simulink model "PTSD_single_channel_local_min_max_2"  (R2019b)
settings: Solver=VariableStepAuto  StartTime=0.0  StopTime=10  RelTol=1e-3
libraries: simulink x10, dspstat3 x7, dspswit3 x1
settings Model: Creator=sbuccelli  LastModifiedBy=sbuccelli

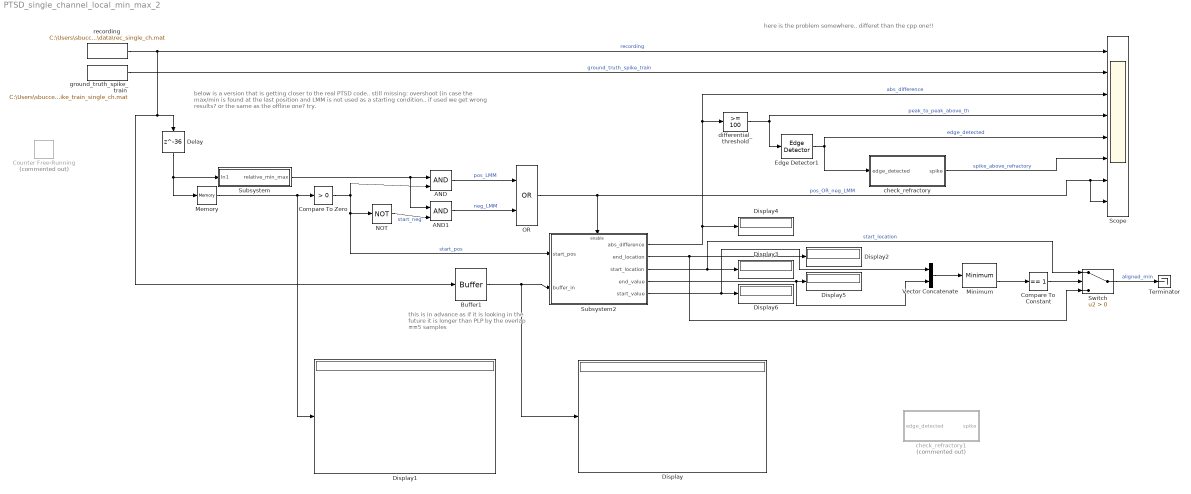
== system PTSD_single_channel_local_min_max_2 ==
  note: here is the problem somewhere.. differet than the cpp one!!
  note: below is a version that is getting closer to the real PTSD code..
      | still missing: overshoot (in case the max/min is found at the last position and LMM is not used as a starting condition.. if used we get wrong results? or the same as the offline one? try.
  note: this is in advance as if it is looking in the future
      | it is longer than PLP by the overlap ==5 samples
  AND : Logic  IconShape=distinctive  AllPortsSameDT=off  OutDataTypeStr=boolean
  AND1 : Logic  IconShape=distinctive  AllPortsSameDT=off  OutDataTypeStr=boolean
  Buffer1 : Buffer  N=38  V=37  OutputFrames=off
  Compare To Constant : simulink/Logic and Bit Operations/Compare To Constant  relop===  const=1  OutDataTypeStr=boolean
  Compare To Zero : simulink/Logic and Bit Operations/Compare To Zero  relop=>  OutDataTypeStr=boolean
  Counter Free-Running : simulink/Sources/Counter Free-Running  Commented=on  NumBits=32  tsamp=-1
  Delay : Delay  DelayLength=36
  Display{,1..6} (7 alike) : Display
  Edge Detector1 : dspswit3/Edge Detector  InputProcessing=Columns as channels (frame based)
      settings: SourceProductName=DSP System Toolbox  SourceProductBaseCode=DS
  Memory : Memory  InheritSampleTime=on
  Minimum : dspstat3/Minimum  operation=minimum  fcn=Value and Index  indexBase=One  operateOver=Each column  Dimension=1  InputProcessing=Columns as channels (frame based)  reset=None  roiEnable=off  roiType=Rectangles  roiPortion=Entire ROI  roiOutput=Individual statistics for each ROI  roiFlag=off  roundingMode=Floor  overflowMode=off
      settings: SourceProductName=DSP System Toolbox  SourceProductBaseCode=DS
  NOT : Logic  Operator=NOT  IconShape=distinctive  AllPortsSameDT=off  OutDataTypeStr=boolean
  OR : Logic  Operator=OR  IconShape=distinctive  AllPortsSameDT=off  OutDataTypeStr=boolean
  Scope : Scope  NumInputPorts=8
  Subsystem : Subsystem
  Subsystem2 : Subsystem
  Switch : Switch  Criteria=u2 > Threshold
  Terminator : Terminator
  Vector Concatenate : Concatenate
  check_refractory : Subsystem
  check_refractory1 : Subsystem  Commented=on
  differential_threshold : simulink/Logic and Bit Operations/Compare To Constant  relop=>=  const=100  OutDataTypeStr=boolean
  ground_truth_spike_train : FromFile  FileName=C:\Users\sbuccelli\Documents\GitHub\closed-loop-neuroscience\data\spike_train_single_ch.mat  SampleTime=1/32e3
  recording : FromFile  FileName=C:\Users\sbuccelli\Documents\GitHub\closed-loop-neuroscience\data\rec_single_ch.mat  SampleTime=1/32e3
  wires:
  recording/1 -> Buffer1/1, Delay/1, Scope/1  "recording"
  ground_truth_spike_train/1 -> Scope/2  "ground_truth_spike_train"
  Subsystem/1(relative_min_max) -> AND/1, AND1/1
  Compare To Zero/1 -> Subsystem2/1(start_pos), NOT/1, AND/2  "start_pos"
  NOT/1 -> AND1/2  "start_neg"
  AND/1 -> OR/1  "pos_LMM"
  AND1/1 -> OR/2  "neg_LMM"
  OR/1 -> Scope/7, Scope/8, Subsystem2/Enable  "pos_OR_neg_LMM"
  Delay/1 -> Memory/1, Subsystem/1(In1)
  differential_threshold/1 -> Scope/4, Edge Detector1/1  "peak_to_peak_above_th"
  Subsystem2/1(abs_difference) -> Display4/1, Scope/3, differential_threshold/1  "abs_difference"
  Buffer1/1 -> Display/1, Subsystem2/2(buffer_in)
  Edge Detector1/1 -> check_refractory/1(edge_detected), Scope/5  "edge_detected"
  check_refractory/1(spike) -> Scope/6  "spike_above_refractory"
  Memory/1 -> Display1/1, Compare To Zero/1
  Subsystem2/2(end_location) -> Switch/3, Display2/1
  Subsystem2/4(end_value) -> Vector Concatenate/2, Display5/1
  Subsystem2/5(start_value) -> Vector Concatenate/1, Display6/1
  Subsystem2/3(start_location) -> Switch/1, Display3/1  "start_location"
  Vector Concatenate/1 -> Minimum/1
  Minimum/2 -> Compare To Constant/1
  Compare To Constant/1 -> Switch/2
  Switch/1 -> Terminator/1  "aligned_min"

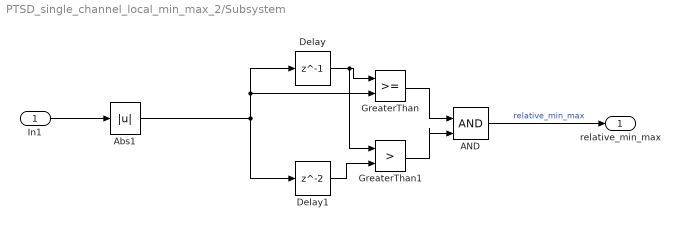
== system PTSD_single_channel_local_min_max_2/Subsystem ==
  In1 : Inport
  AND : Logic  IconShape=distinctive  AllPortsSameDT=off  OutDataTypeStr=boolean
  Abs1 : Abs
  Delay : Delay  DelayLength=1
  Delay1 : Delay
  GreaterThan : RelationalOperator  OutDataTypeStr=boolean  RndMeth=Simplest
  GreaterThan1 : RelationalOperator  Operator=>  OutDataTypeStr=boolean  RndMeth=Simplest
  relative_min_max : Outport
  wires:
  In1/1 -> Abs1/1
  Delay1/1 -> GreaterThan1/2
  GreaterThan1/1 -> AND/2
  GreaterThan/1 -> AND/1
  Delay/1 -> GreaterThan1/1, GreaterThan/1
  AND/1 -> relative_min_max/1  "relative_min_max"
  Abs1/1 -> Delay/1, GreaterThan/2, Delay1/1

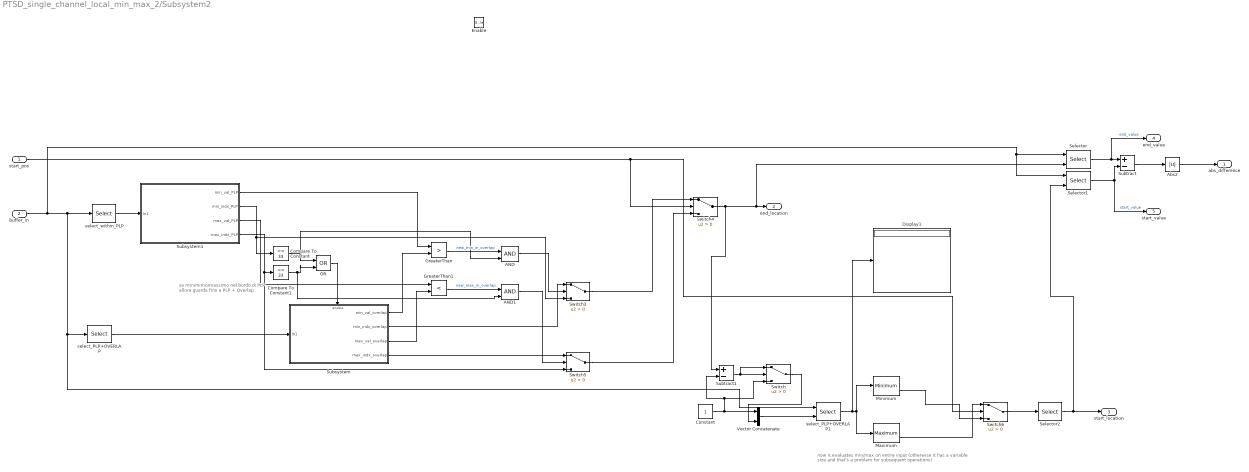
== system PTSD_single_channel_local_min_max_2/Subsystem2 ==
  note: now it evaluates min/max on entire input (otherwise it has a variable size and that's a problem for subsequent operations)
  note: se minimimo/massimo nel bordo di PLP allora guarda fino a PLP + Overlap
  start_pos : Inport
  buffer_in : Inport  Port=2
  Enable : EnablePort  PropagateVarSize=During execution
  AND : Logic  IconShape=distinctive  AllPortsSameDT=off  OutDataTypeStr=boolean
  AND1 : Logic  IconShape=distinctive  AllPortsSameDT=off  OutDataTypeStr=boolean
  Abs2 : Abs
  Compare To Constant : simulink/Logic and Bit Operations/Compare To Constant  relop===  const=33  OutDataTypeStr=boolean
  Compare To Constant1 : simulink/Logic and Bit Operations/Compare To Constant  relop===  const=33  OutDataTypeStr=boolean
  Constant : Constant
  Display1 : Display
  GreaterThan : RelationalOperator  Operator=>  OutDataTypeStr=boolean  RndMeth=Simplest
  GreaterThan1 : RelationalOperator  Operator=<  OutDataTypeStr=boolean  RndMeth=Simplest
  Maximum : dspstat3/Maximum  operation=maximum  fcn=Value and Index  indexBase=One  operateOver=Entire input  Dimension=1  InputProcessing=Columns as channels (frame based)  reset=None  roiEnable=off  roiType=Rectangles  roiPortion=Entire ROI  roiOutput=Individual statistics for each ROI  roiFlag=off  roundingMode=Floor  overflowMode=off  accumDataTypeStr=Inherit: Same as product output  accumLastDataTypeStr=Inherit: Same as product output
  Minimum : dspstat3/Minimum  operation=minimum  fcn=Value and Index  indexBase=One  operateOver=Entire input  Dimension=1  InputProcessing=Columns as channels (frame based)  reset=None  roiEnable=off  roiType=Rectangles  roiPortion=Entire ROI  roiOutput=Individual statistics for each ROI  roiFlag=off  roundingMode=Floor  overflowMode=off
      settings: SourceProductName=DSP System Toolbox  SourceProductBaseCode=DS
  OR : Logic  Operator=OR  IconShape=distinctive  AllPortsSameDT=off  OutDataTypeStr=boolean
  Selector : Selector  IndexOptions=Index vector (port)  Indices=[1 3]  OutputSizes=1
  Selector1 : Selector  IndexOptions=Index vector (port)  Indices=[1 3]  OutputSizes=1
  Selector2 : Selector  NumberOfDimensions=2  IndexOptions=Select all,Index vector (dialog)  Indices=[1 3],1  OutputSizes=1,1
  Subsystem : Subsystem
  Subsystem1 : Subsystem
  Subtract : Sum  Inputs=+-
  Subtract1 : Sum  Inputs=+-
  Switch{,3..6} (5 alike) : Switch  Criteria=u2 > Threshold
  Vector Concatenate : Concatenate
  select_PLP+OVERLAP : Selector  NumberOfDimensions=2  InputPortWidth=3  IndexOptions=Index vector (dialog),Index vector (dialog)  Indices=[34:38],1  OutputSizes=1,1
  select_PLP+OVERLAP1 : Selector  NumberOfDimensions=2  InputPortWidth=3  IndexOptions=Starting and ending indices (port),Index vector (dialog)  Indices=[25:29],1  OutputSizes=1,1
  select_within_PLP : Selector  NumberOfDimensions=2  InputPortWidth=3  IndexOptions=Index vector (dialog),Index vector (dialog)  Indices=[1:33],1  OutputSizes=1,1
  abs_difference : Outport
  end_location : Outport  Port=2
  start_location : Outport  Port=3
  end_value : Outport  Port=4
  start_value : Outport  Port=5
  wires:
  Abs2/1 -> abs_difference/1
  buffer_in/1 -> Selector1/1, Selector/1, select_within_PLP/1, select_PLP+OVERLAP1/1, select_PLP+OVERLAP/1
  Subtract/1 -> Abs2/1
  Compare To Constant/1 -> OR/1, AND/2
  Compare To Constant1/1 -> AND1/2, OR/2
  OR/1 -> Subsystem/Enable
  select_PLP+OVERLAP/1 -> Subsystem/1(In1)
  select_within_PLP/1 -> Subsystem1/1(In1)
  Subsystem1/2(min_indx_PLP) -> Switch3/3, Compare To Constant/1
  Subsystem1/4(max_indx_PLP) -> Switch5/3, Compare To Constant1/1
  Subsystem1/1(min_val_PLP) -> GreaterThan/1
  Subsystem/1(min_val_overlap) -> GreaterThan/2
  Subsystem1/3(max_val_PLP) -> GreaterThan1/1
  Subsystem/3(max_val_overlap) -> GreaterThan1/2
  GreaterThan/1 -> AND/1  "new_min_in_overlap"
  GreaterThan1/1 -> AND1/1  "new_max_in_overlap"
  AND/1 -> Switch3/2
  AND1/1 -> Switch5/2
  Switch3/1 -> Switch4/1
  Switch5/1 -> Switch4/3
  Subsystem/2(min_indx_overlap) -> Switch3/1
  Subsystem/4(max_indx_overlap) -> Switch5/1
  Vector Concatenate/1 -> select_PLP+OVERLAP1/2
  start_pos/1 -> Switch4/2, Switch6/2
  select_PLP+OVERLAP1/1 -> Display1/1, Maximum/1, Minimum/1
  Minimum/2 -> Switch6/3
  Maximum/2 -> Switch6/1
  Selector/1 -> end_value/1, Subtract/1  "end_value"
  Selector1/1 -> start_value/1, Subtract/2  "start_value"
  Switch4/1 -> Selector/2, end_location/1, Subtract1/1
  Switch6/1 -> Selector2/1
  Selector2/1 -> start_location/1, Selector1/2
  Subtract1/1 -> Switch/1, Switch/2
  Constant/1 -> Vector Concatenate/1, Switch/3, Subtract1/2
  Switch/1 -> Vector Concatenate/2

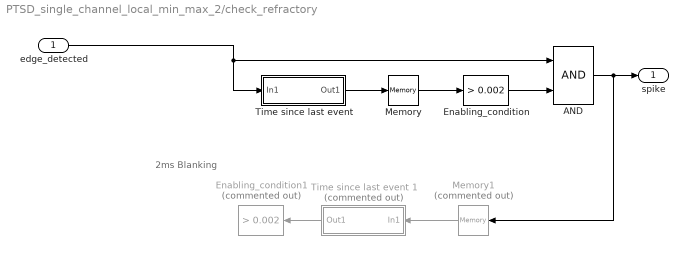
== system PTSD_single_channel_local_min_max_2/check_refractory ==
  note: 2ms Blanking
  edge_detected : Inport
  AND : Logic  IconShape=distinctive  AllPortsSameDT=off  OutDataTypeStr=boolean
  Enabling_condition : simulink/Logic and Bit Operations/Compare To Constant  relop=>  const=0.002  OutDataTypeStr=boolean
  Enabling_condition1 : simulink/Logic and Bit Operations/Compare To Constant  Commented=on  relop=>  const=0.002  OutDataTypeStr=boolean
  Memory : Memory  InheritSampleTime=on
  Memory1 : Memory  Commented=on  InheritSampleTime=on
  "Time since last event " : Subsystem
  Time since last event 1 : Subsystem  Commented=on
  spike : Outport
  wires:
  Enabling_condition/1 -> AND/2
  Memory/1 -> Enabling_condition/1
  "Time since last event "/1(Out1) -> Memory/1
  AND/1 -> Memory1/1, spike/1
  Time since last event 1/1(Out1) -> Enabling_condition1/1
  edge_detected/1 -> "Time since last event "/1(In1), AND/1
  Memory1/1 -> Time since last event 1/1(In1)

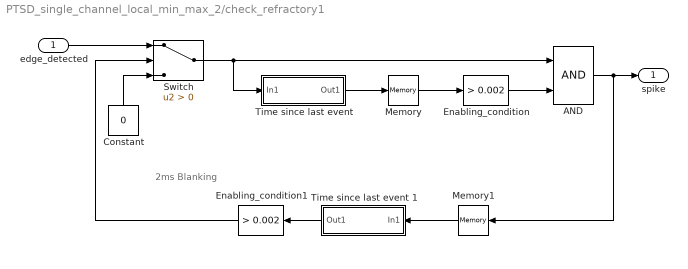
== system PTSD_single_channel_local_min_max_2/check_refractory1 ==
  note: 2ms Blanking
  edge_detected : Inport
  AND : Logic  IconShape=distinctive  AllPortsSameDT=off  OutDataTypeStr=boolean
  Constant : Constant  Value=0  SampleTime=-1
  Enabling_condition : simulink/Logic and Bit Operations/Compare To Constant  relop=>  const=0.002  OutDataTypeStr=boolean
  Enabling_condition1 : simulink/Logic and Bit Operations/Compare To Constant  relop=>  const=0.002  OutDataTypeStr=boolean
  Memory : Memory  InheritSampleTime=on
  Memory1 : Memory  InheritSampleTime=on
  Switch : Switch  Criteria=u2 > Threshold
  "Time since last event " : Subsystem
  Time since last event 1 : Subsystem
  spike : Outport
  wires:
  Enabling_condition/1 -> AND/2
  Memory/1 -> Enabling_condition/1
  "Time since last event "/1(Out1) -> Memory/1
  AND/1 -> Memory1/1, spike/1
  Time since last event 1/1(Out1) -> Enabling_condition1/1
  edge_detected/1 -> Switch/1
  Constant/1 -> Switch/3
  Switch/1 -> "Time since last event "/1(In1), AND/1
  Memory1/1 -> Time since last event 1/1(In1)
  Enabling_condition1/1 -> Switch/2

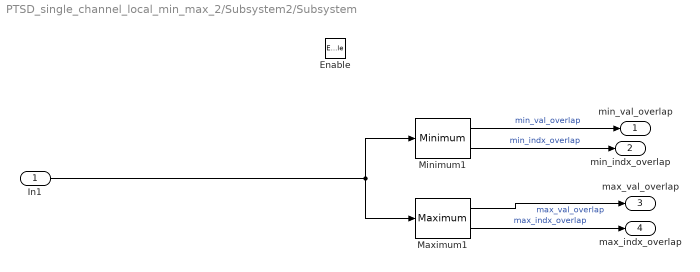
== system PTSD_single_channel_local_min_max_2/Subsystem2/Subsystem ==
  In1 : Inport
  Enable : EnablePort
  Maximum1 : dspstat3/Maximum  operation=maximum  fcn=Value and Index  indexBase=One  operateOver=Each column  Dimension=1  InputProcessing=Columns as channels (frame based)  reset=None  roiEnable=off  roiType=Rectangles  roiPortion=Entire ROI  roiOutput=Individual statistics for each ROI  roiFlag=off  roundingMode=Floor  overflowMode=off  accumDataTypeStr=Inherit: Same as product output  accumLastDataTypeStr=Inherit: Same as product output
  Minimum1 : dspstat3/Minimum  operation=minimum  fcn=Value and Index  indexBase=One  operateOver=Each column  Dimension=1  InputProcessing=Columns as channels (frame based)  reset=None  roiEnable=off  roiType=Rectangles  roiPortion=Entire ROI  roiOutput=Individual statistics for each ROI  roiFlag=off  roundingMode=Floor  overflowMode=off
      settings: SourceProductName=DSP System Toolbox  SourceProductBaseCode=DS
  min_val_overlap : Outport
  min_indx_overlap : Outport  Port=2
  max_val_overlap : Outport  Port=3
  max_indx_overlap : Outport  Port=4
  wires:
  Minimum1/2 -> min_indx_overlap/1  "min_indx_overlap"
  In1/1 -> Minimum1/1, Maximum1/1
  Maximum1/2 -> max_indx_overlap/1  "max_indx_overlap"
  Minimum1/1 -> min_val_overlap/1  "min_val_overlap"
  Maximum1/1 -> max_val_overlap/1  "max_val_overlap"

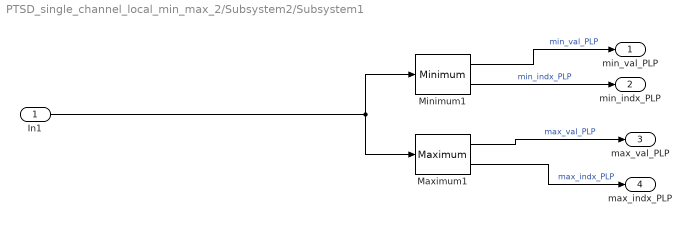
== system PTSD_single_channel_local_min_max_2/Subsystem2/Subsystem1 ==
  In1 : Inport
  Maximum1 : dspstat3/Maximum  operation=maximum  fcn=Value and Index  indexBase=One  operateOver=Each column  Dimension=1  InputProcessing=Columns as channels (frame based)  reset=None  roiEnable=off  roiType=Rectangles  roiPortion=Entire ROI  roiOutput=Individual statistics for each ROI  roiFlag=off  roundingMode=Floor  overflowMode=off  accumDataTypeStr=Inherit: Same as product output  accumLastDataTypeStr=Inherit: Same as product output
  Minimum1 : dspstat3/Minimum  operation=minimum  fcn=Value and Index  indexBase=One  operateOver=Each column  Dimension=1  InputProcessing=Columns as channels (frame based)  reset=None  roiEnable=off  roiType=Rectangles  roiPortion=Entire ROI  roiOutput=Individual statistics for each ROI  roiFlag=off  roundingMode=Floor  overflowMode=off
      settings: SourceProductName=DSP System Toolbox  SourceProductBaseCode=DS
  min_val_PLP : Outport
  min_indx_PLP : Outport  Port=2
  max_val_PLP : Outport  Port=3
  max_indx_PLP : Outport  Port=4
  wires:
  Minimum1/2 -> min_indx_PLP/1  "min_indx_PLP"
  In1/1 -> Minimum1/1, Maximum1/1
  Maximum1/2 -> max_indx_PLP/1  "max_indx_PLP"
  Minimum1/1 -> min_val_PLP/1  "min_val_PLP"
  Maximum1/1 -> max_val_PLP/1  "max_val_PLP"

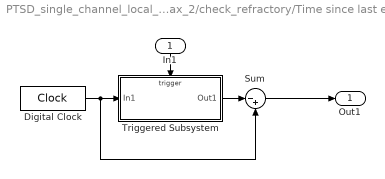
== system PTSD_single_channel_local_min_max_2/check_refractory/Time since last event  ==
  In1 : Inport
  Digital Clock : DigitalClock  SampleTime=1/32e3
  Sum : Sum  Inputs=|-+
  Triggered Subsystem : Subsystem  TreatAsAtomicUnit=on
  Out1 : Outport
  wires:
  Digital Clock/1 -> Sum/2, Triggered Subsystem/1(In1)
  Triggered Subsystem/1(Out1) -> Sum/1
  In1/1 -> Triggered Subsystem/Trigger
  Sum/1 -> Out1/1

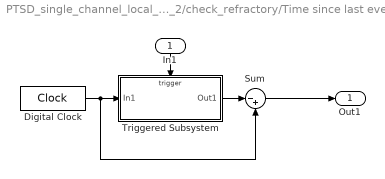
== system PTSD_single_channel_local_min_max_2/check_refractory/Time since last event 1 ==
  In1 : Inport
  Digital Clock : DigitalClock  SampleTime=1/32e3
  Sum : Sum  Inputs=|-+
  Triggered Subsystem : Subsystem  TreatAsAtomicUnit=on
  Out1 : Outport
  wires:
  Digital Clock/1 -> Sum/2, Triggered Subsystem/1(In1)
  Triggered Subsystem/1(Out1) -> Sum/1
  In1/1 -> Triggered Subsystem/Trigger
  Sum/1 -> Out1/1

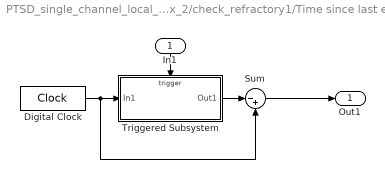
== system PTSD_single_channel_local_min_max_2/check_refractory1/Time since last event  ==
  In1 : Inport
  Digital Clock : DigitalClock  SampleTime=1/32e3
  Sum : Sum  Inputs=|-+
  Triggered Subsystem : Subsystem  TreatAsAtomicUnit=on
  Out1 : Outport
  wires:
  Digital Clock/1 -> Sum/2, Triggered Subsystem/1(In1)
  Triggered Subsystem/1(Out1) -> Sum/1
  In1/1 -> Triggered Subsystem/Trigger
  Sum/1 -> Out1/1

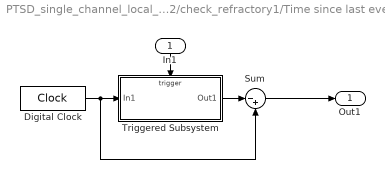
== system PTSD_single_channel_local_min_max_2/check_refractory1/Time since last event 1 ==
  In1 : Inport
  Digital Clock : DigitalClock  SampleTime=1/32e3
  Sum : Sum  Inputs=|-+
  Triggered Subsystem : Subsystem  TreatAsAtomicUnit=on
  Out1 : Outport
  wires:
  Digital Clock/1 -> Sum/2, Triggered Subsystem/1(In1)
  Triggered Subsystem/1(Out1) -> Sum/1
  In1/1 -> Triggered Subsystem/Trigger
  Sum/1 -> Out1/1

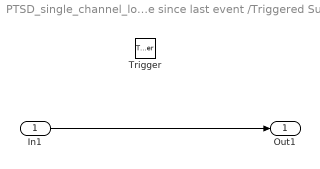
== system PTSD_single_channel_local_min_max_2/check_refractory/Time since last event /Triggered Subsystem ==
  In1 : Inport
  Trigger : TriggerPort  VariantControl=Variant
  Out1 : Outport
  wires:
  In1/1 -> Out1/1

== system PTSD_single_channel_local_min_max_2/check_refractory/Time since last event 1/Triggered Subsystem ==
  In1 : Inport
  Trigger : TriggerPort  VariantControl=Variant
  Out1 : Outport
  wires:
  In1/1 -> Out1/1

== system PTSD_single_channel_local_min_max_2/check_refractory1/Time since last event /Triggered Subsystem ==
  In1 : Inport
  Trigger : TriggerPort  VariantControl=Variant
  Out1 : Outport
  wires:
  In1/1 -> Out1/1

== system PTSD_single_channel_local_min_max_2/check_refractory1/Time since last event 1/Triggered Subsystem ==
  In1 : Inport
  Trigger : TriggerPort  VariantControl=Variant
  Out1 : Outport
  wires:
  In1/1 -> Out1/1
